simulink model "systemID"  (R2017b)
settings: Solver=FixedStepAuto  StartTime=0.0  StopTime=50  FixedStep=0.01  RelTol=1e-3
undefined symbols (not defined in the file): CoordinateFrame, TypeMask, Velocity
libraries: robotlib x3
settings Model: Creator=bshang2  LastModifiedBy=bshang2

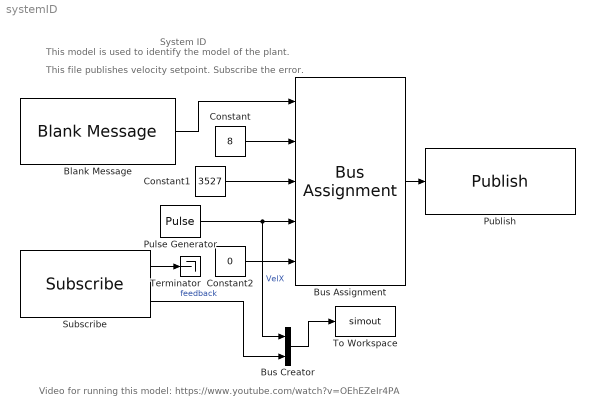
== system systemID ==
  note: Video for running this model: https://www.youtube.com/watch?v=OEhEZeIr4PA
  note: System ID
  note: This file publishes velocity setpoint. Subscribe the error.
  note: This model is used to identify the model of the plant.
  Blank Message : robotlib/Blank Message  SourceLibraryInfo=This block requires Robotics System Toolbox  messageType=mavros_msgs/PositionTarget  SampleTime=inf
      settings: SourceProductBaseCode=RO
  Bus Assignment : BusAssignment  AssignedSignals=CoordinateFrame,TypeMask,Velocity.X,Velocity.Y
  Bus Creator : BusCreator  Inputs=2
  Constant : Constant  Value=8  OutDataTypeStr=uint8
  Constant1 : Constant  Value=3527  OutDataTypeStr=uint16
  Constant2 : Constant  Value=0
  Publish : robotlib/Publish  SourceLibraryInfo=This block requires Robotics System Toolbox  topicSource=Specify your own  topic=/mavros/setpoint_raw/local  messageType=mavros_msgs/PositionTarget  messageQueueLength=1
      settings: SourceProductBaseCode=RO
  Pulse Generator : DiscretePulseGenerator  PulseType=Time based  Amplitude=-0.1  Period=5  PulseWidth=25  SampleTime=0
  Subscribe : robotlib/Subscribe  SourceLibraryInfo=This block requires Robotics System Toolbox  topicSource=Select from ROS network  topic=/matlab/err  messageType=geometry_msgs/Pose2D  sampleTime=-1  messageQueueLength=1
      settings: SourceProductBaseCode=RO
  Terminator : Terminator
  To Workspace : ToWorkspace  VariableName=simout  SaveFormat=Timeseries  SampleTime=-1
  wires:
  Blank Message/1 -> Bus Assignment/1
  Bus Assignment/1 -> Publish/1
  Constant/1 -> Bus Assignment/2
  Constant1/1 -> Bus Assignment/3
  Constant2/1 -> Bus Assignment/5
  Pulse Generator/1 -> Bus Creator/1, Bus Assignment/4  "VelX"
  Subscribe/1 -> Terminator/1
  Subscribe/2 -> Bus Creator/2  "feedback"
  Bus Creator/1 -> To Workspace/1
